simulink model "calculation_of_Inductor"  (R2024a)
settings: Solver=VariableStepAuto  StartTime=0.0  StopTime=10.0  RelTol=1e-3
settings Model: Creator=Lenovo  LastModifiedBy=Lenovo

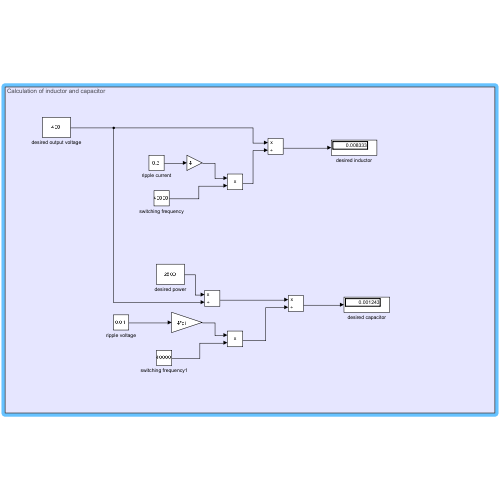
[thumbnail: Simulink's stored preview of the top-level diagram]
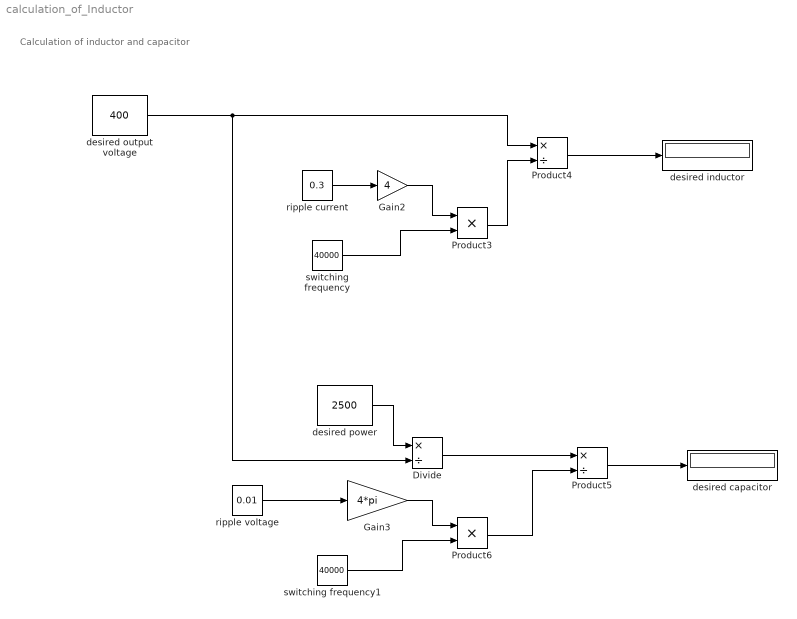
== system calculation_of_Inductor ==
  note: Calculation of inductor and capacitor
  Divide : Product  Inputs=*/
  Gain2 : Gain  Gain=4
  Gain3 : Gain  Gain=4*pi
  Product3 : Product
  Product4 : Product  Inputs=*/
  Product5 : Product  Inputs=*/
  Product6 : Product
  desired capacitor : Display
  desired inductor : Display
  desired output voltage : Constant  Value=400
  desired power : Constant  Value=2500
  ripple current : Constant  Value=0.3
  ripple voltage : Constant  Value=0.01
  switching frequency : Constant  Value=40000
  switching frequency1 : Constant  Value=40000
  wires:
  switching frequency/1 -> Product3/2
  Gain3/1 -> Product6/1
  Product6/1 -> Product5/2
  ripple current/1 -> Gain2/1
  Product5/1 -> desired capacitor/1
  Product4/1 -> desired inductor/1
  switching frequency1/1 -> Product6/2
  ripple voltage/1 -> Gain3/1
  Divide/1 -> Product5/1
  desired output voltage/1 -> Divide/2, Product4/1
  Product3/1 -> Product4/2
  desired power/1 -> Divide/1
  Gain2/1 -> Product3/1
